simulink model "myTHD_test"  (R2024a)
settings: Solver=VariableStepAuto  StartTime=0.0  StopTime=2  RelTol=1e-3
undefined symbols (not defined in the file or in its folder): BUFFER_LEN, SAMPLING_FREQ, signal_1
libraries: hdlsllib x1, dsphdlxfrm2 x1, dspsrcs4 x1
settings Model: Creator=Jan Rosa  LastModifiedBy=Jan Rosa

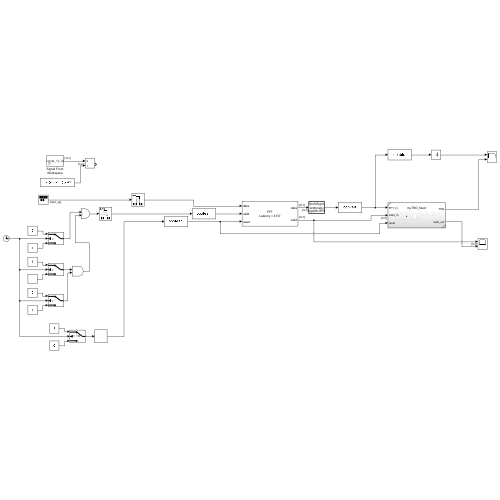
[thumbnail: Simulink's stored preview of the top-level diagram]
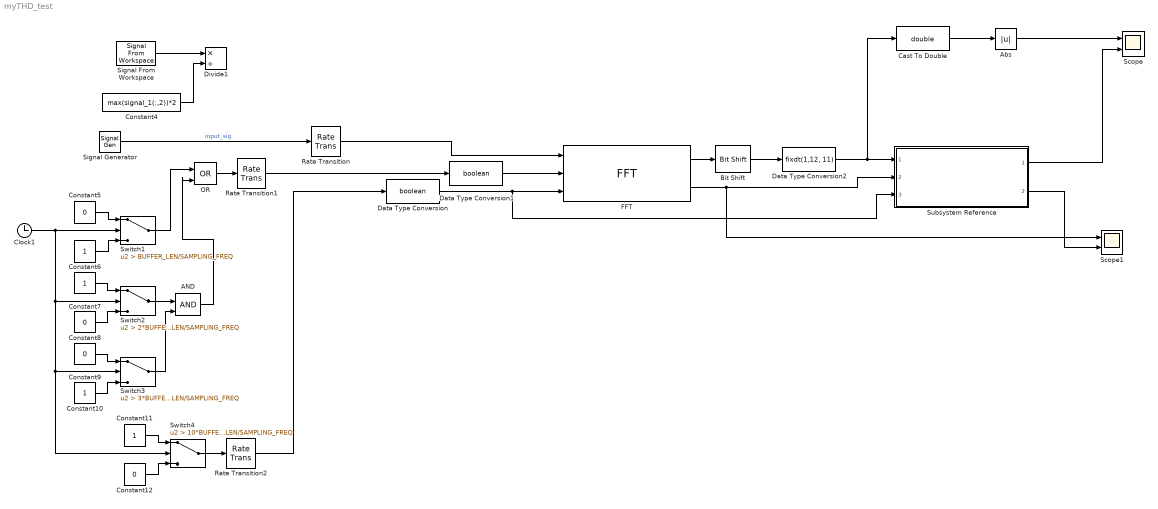
== system myTHD_test ==
  AND : Logic  IconShape=distinctive  AllPortsSameDT=off  OutDataTypeStr=boolean
  Abs : Abs  SaturateOnIntegerOverflow=off
  Bit Shift : hdlsllib/Logic and Bit Operations/Bit Shift  mode=Shift Right Arithmetic  N=log2(BUFFER_LEN)
  Cast To Double : DataTypeConversion  OutDataTypeStr=double  SaturateOnIntegerOverflow=off  RndMeth=Floor
  Clock1 : Clock
  Constant{6..7,10..11} (4 alike) : Constant
  Constant{5,8..9,12} (4 alike) : Constant  Value=0
  Constant4 : Constant  Value=max(signal_1(:,2))*2
  Data Type Conversion : DataTypeConversion  OutDataTypeStr=boolean  SaturateOnIntegerOverflow=off  RndMeth=Floor
  Data Type Conversion1 : DataTypeConversion  OutDataTypeStr=boolean  SaturateOnIntegerOverflow=off  RndMeth=Floor
  Data Type Conversion2 : DataTypeConversion  OutDataTypeStr=fixdt(1,12, 11)  SaturateOnIntegerOverflow=off  RndMeth=Floor
  Divide1 : Product  Inputs=*/
  FFT : dsphdlxfrm2/FFT  Architecture=Streaming Radix 2^2  FFTLengthSource=Property  FFTLength=BUFFER_LEN  FFTLengthMax=1024  ComplexMultiplication=Use 3 multipliers and 5 adders  BitReversedOutput=off  BitReversedInput=off  Normalize=off  SimulateUsing=Code generation  RoundingMethod=Floor  ResetInputPort=on  StartOutputPort=off  EndOutputPort=off
  OR : Logic  Operator=OR  IconShape=distinctive  AllPortsSameDT=off  OutDataTypeStr=boolean
  Rate Transition : RateTransition  Deterministic=off  OutPortSampleTime=1/SAMPLING_FREQ
  Rate Transition1 : RateTransition  OutPortSampleTime=1/SAMPLING_FREQ
  Rate Transition2 : RateTransition  OutPortSampleTime=1/SAMPLING_FREQ
  Scope : Scope  NumInputPorts=2
  Scope1 : Scope  NumInputPorts=2
  Signal Generator : SignalGenerator  WaveForm=square  Amplitude=0.49999  Frequency=50
  Signal From Workspace : dspsrcs4/Signal From Workspace  X=signal_1(:, 2)  Ts=signal_1(2, 1)  nsamps=1  OutputAfterFinalValue=Cyclic repetition  ignoreOrWarnInputAndFrameLengths=off  OutputFrames=off
  Subsystem Reference : Subsystem  ReferencedSubsystem=myTHD_fixed
  Switch1 : Switch  Criteria=u2 > Threshold  Threshold=BUFFER_LEN/SAMPLING_FREQ  SaturateOnIntegerOverflow=off  InputSameDT=off
  Switch2 : Switch  Criteria=u2 > Threshold  Threshold=2*BUFFER_LEN/SAMPLING_FREQ  SaturateOnIntegerOverflow=off  InputSameDT=off
  Switch3 : Switch  Criteria=u2 > Threshold  Threshold=3*BUFFER_LEN/SAMPLING_FREQ  SaturateOnIntegerOverflow=off  InputSameDT=off
  Switch4 : Switch  Criteria=u2 > Threshold  Threshold=10*BUFFER_LEN/SAMPLING_FREQ  SaturateOnIntegerOverflow=off  InputSameDT=off
  wires:
  Rate Transition1/1 -> Data Type Conversion1/1
  Rate Transition2/1 -> Data Type Conversion/1
  Rate Transition/1 -> FFT/1
  Data Type Conversion1/1 -> FFT/2
  Data Type Conversion/1 -> Subsystem Reference/3, FFT/3
  FFT/2 -> Scope1/1, Subsystem Reference/2
  Subsystem Reference/2 -> Scope1/2
  Bit Shift/1 -> Data Type Conversion2/1
  Abs/1 -> Scope/1
  Subsystem Reference/1 -> Scope/2
  Constant4/1 -> Divide1/2
  Signal From Workspace/1 -> Divide1/1
  Constant10/1 -> Switch3/3
  Switch2/1 -> AND/1
  Clock1/1 -> Switch3/2, Switch4/2, Switch2/2, Switch1/2
  Constant12/1 -> Switch4/3
  AND/1 -> OR/2
  Constant11/1 -> Switch4/1
  Constant9/1 -> Switch3/1
  Switch1/1 -> OR/1
  Constant6/1 -> Switch1/3
  Constant7/1 -> Switch2/1
  Constant5/1 -> Switch1/1
  Switch3/1 -> AND/2
  Constant8/1 -> Switch2/3
  Switch4/1 -> Rate Transition2/1
  OR/1 -> Rate Transition1/1
  Signal Generator/1 -> Rate Transition/1  "input_sig"
  FFT/1 -> Bit Shift/1
  Data Type Conversion2/1 -> Cast To Double/1, Subsystem Reference/1
  Cast To Double/1 -> Abs/1
